simulink model "QuadcopterController"  (R2019a)
settings: Solver=VariableStepAuto  StartTime=0.0  StopTime=50  RelTol=1e-3
InitFcn:
  | parameters
values from neighbouring files (symbols this model uses):
  attitudeInit = [0;0;0]    [parameters.m]
  b = 5.9347e-06    [parameters.m]
  d = 1.2181e-07    [parameters.m]
  g = 9.81    [parameters.m]
  I = diag([Ix,Iy,Iz])    [parameters.m]
  Ix = 0.0073    [parameters.m]
  Iy = 0.0073    [parameters.m]
  Iz = 0.0117    [parameters.m]
  ks = 735    [parameters.m]
  Kth = b*lambda    [parameters.m]
  kxih = 0.7    [parameters.m]
  L = 0.17    [parameters.m]
  lambda = w0^2/u0    [parameters.m]
  m = 0.616    [parameters.m]
  omegaInit = [0;0;0]    [parameters.m]
  posInit = [0;0;0]    [parameters.m]
  tau = 1/200    (= 0.005)    [parameters.m]
  u0 = 0.49    [parameters.m]
  velInit = [0;0;0]    [parameters.m]
  w_n = 8    [parameters.m]
  wh_n = 2    [parameters.m]
  zeta = 0.7    [parameters.m]
settings Model: Creator=NGUYEN  LastModifiedBy=ASUS
settings SolverCC: ZeroCrossAlgorithm=Adaptive
settings OptimizationCC: LifeSpan=inf
settings DebuggingCC: IgnoredZcDiagnostic=none  ArithmeticOperatorsInVariantConditions=warning
settings CodeAppCC: StateflowObjectComments=on

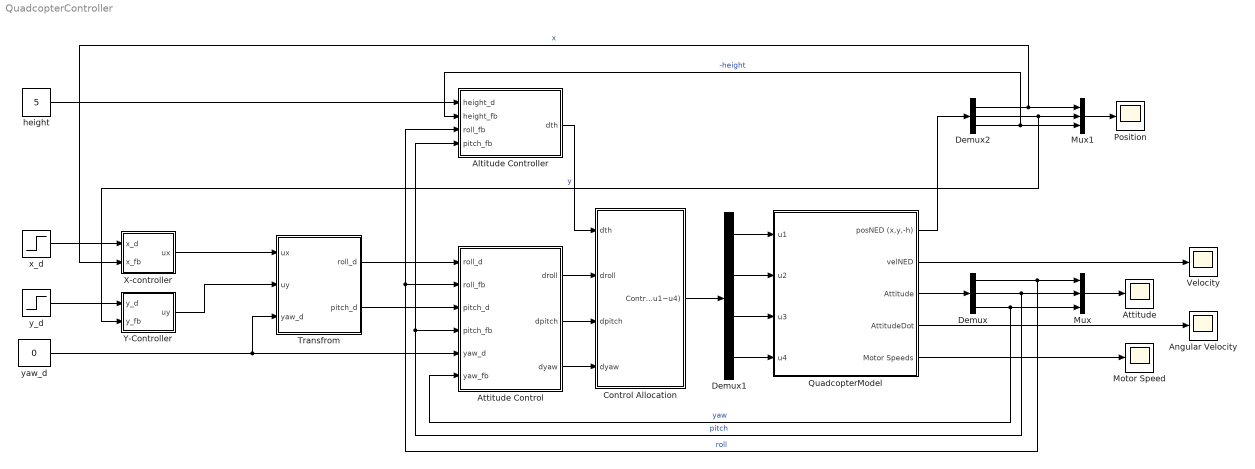
== system QuadcopterController ==
  Altitude Controller : Subsystem
  Angular Velocity : Scope
  Attitude : Scope
  Attitude Control : Subsystem
  Control Allocation : Subsystem
  Demux : Demux  Outputs=3
  Demux1 : Demux
  Demux2 : Demux  Outputs=3
  Motor Speed : Scope
  Mux : Mux  Inputs=3
  Mux1 : Mux  Inputs=3
  Position : Scope
  QuadcopterModel : Subsystem
  Transfrom : Subsystem
  Velocity : Scope
  X-controller : Subsystem
  Y-Controller : Subsystem
  height : Constant  Value=5
  x_d : Step  Time=0  After=5  SampleTime=0
  y_d : Step  Time=0  After=7  SampleTime=0
  yaw_d : Constant  Value=0
  wires:
  Demux/1 -> Mux/1, Altitude Controller/3(roll_fb), Attitude Control/2(roll_fb)  "roll"
  Demux/2 -> Mux/2, Altitude Controller/4(pitch_fb), Attitude Control/4(pitch_fb)  "pitch"
  Demux/3 -> Mux/3, Attitude Control/6(yaw_fb)  "yaw"
  Demux2/1 -> Mux1/1, X-controller/2(x_fb)  "x"
  Demux2/2 -> Mux1/2, Y-Controller/2(y_fb)  "y"
  Demux2/3 -> Mux1/3, Altitude Controller/2(height_fb)  "-height"
  Mux1/1 -> Position/1
  Mux/1 -> Attitude/1
  height/1 -> Altitude Controller/1(height_d)
  yaw_d/1 -> Attitude Control/5(yaw_d), Transfrom/3(yaw_d)
  X-controller/1(ux) -> Transfrom/1(ux)
  Y-Controller/1(uy) -> Transfrom/2(uy)
  y_d/1 -> Y-Controller/1(y_d)
  x_d/1 -> X-controller/1(x_d)
  Transfrom/1(roll_d) -> Attitude Control/1(roll_d)
  Transfrom/2(pitch_d) -> Attitude Control/3(pitch_d)
  Altitude Controller/1(dth) -> Control Allocation/1(dth)
  Attitude Control/1(droll) -> Control Allocation/2(droll)
  Attitude Control/2(dpitch) -> Control Allocation/3(dpitch)
  Attitude Control/3(dyaw) -> Control Allocation/4(dyaw)
  Control Allocation/1(Controller (u1~u4)) -> Demux1/1
  QuadcopterModel/1(posNED (x,y,-h)) -> Demux2/1
  QuadcopterModel/3(Attitude) -> Demux/1
  Demux1/1 -> QuadcopterModel/1(u1)
  Demux1/2 -> QuadcopterModel/2(u2)
  Demux1/3 -> QuadcopterModel/3(u3)
  Demux1/4 -> QuadcopterModel/4(u4)
  QuadcopterModel/4(AttitudeDot) -> Angular Velocity/1
  QuadcopterModel/2(velNED) -> Velocity/1
  QuadcopterModel/5(Motor Speeds) -> Motor Speed/1

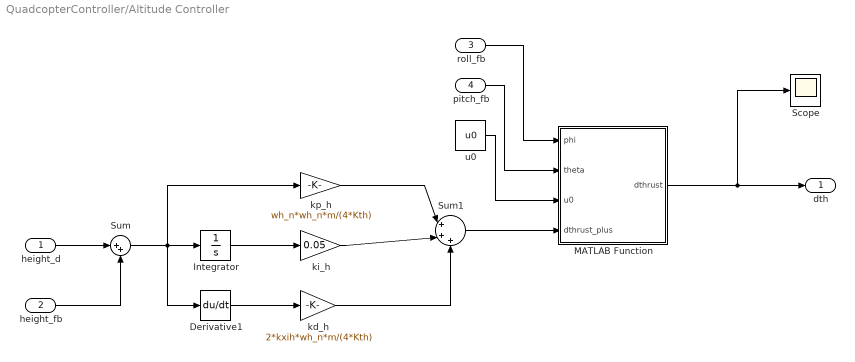
== system QuadcopterController/Altitude Controller ==
  height_d : Inport
  height_fb : Inport  Port=2
  roll_fb : Inport  Port=3
  pitch_fb : Inport  Port=4
  Derivative1 : Derivative
  Integrator : Integrator
  MATLAB Function : MATLAB Function  TreatAsAtomicUnit=on
  Scope : Scope
  Sum : Sum  Inputs=|++
  Sum1 : Sum  Inputs=|+++
  kd_h : Gain  Gain=2*kxih*wh_n*m/(4*Kth)
  ki_h : Gain  Gain=0.05
  kp_h : Gain  Gain=wh_n*wh_n*m/(4*Kth)
  u0 : Constant  Value=u0
  dth : Outport
  wires:
  Derivative1/1 -> kd_h/1
  height_d/1 -> Sum/1
  Sum/1 -> kp_h/1, Integrator/1, Derivative1/1
  height_fb/1 -> Sum/2
  Integrator/1 -> ki_h/1
  ki_h/1 -> Sum1/2
  kp_h/1 -> Sum1/1
  kd_h/1 -> Sum1/3
  Sum1/1 -> MATLAB Function/4(dthrust_plus)
  roll_fb/1 -> MATLAB Function/1(phi)
  pitch_fb/1 -> MATLAB Function/2(theta)
  MATLAB Function/1(dthrust) -> Scope/1, dth/1
  u0/1 -> MATLAB Function/3(u0)

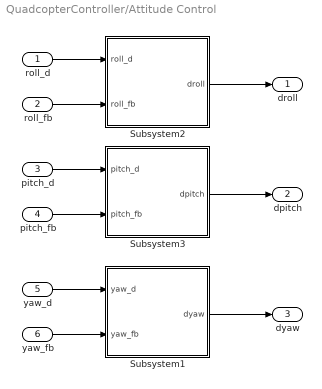
== system QuadcopterController/Attitude Control ==
  roll_d : Inport
  roll_fb : Inport  Port=2
  pitch_d : Inport  Port=3
  pitch_fb : Inport  Port=4
  yaw_d : Inport  Port=5
  yaw_fb : Inport  Port=6
  Subsystem1 : Subsystem
  Subsystem2 : Subsystem
  Subsystem3 : Subsystem
  droll : Outport
  dpitch : Outport  Port=2
  dyaw : Outport  Port=3
  wires:
  roll_d/1 -> Subsystem2/1(roll_d)
  Subsystem3/1(dpitch) -> dpitch/1
  roll_fb/1 -> Subsystem2/2(roll_fb)
  yaw_d/1 -> Subsystem1/1(yaw_d)
  Subsystem2/1(droll) -> droll/1
  pitch_d/1 -> Subsystem3/1(pitch_d)
  pitch_fb/1 -> Subsystem3/2(pitch_fb)
  yaw_fb/1 -> Subsystem1/2(yaw_fb)
  Subsystem1/1(dyaw) -> dyaw/1

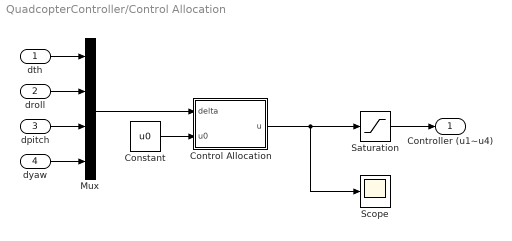
== system QuadcopterController/Control Allocation ==
  dth : Inport
  droll : Inport  Port=2
  dpitch : Inport  Port=3
  dyaw : Inport  Port=4
  Constant : Constant  Value=u0
  Control Allocation : MATLAB Function  TreatAsAtomicUnit=on
  Mux : Mux
  Saturation : Saturate  UpperLimit=1  LowerLimit=0  ZeroCross=off
  Scope : Scope
  Controller (u1~u4) : Outport
  wires:
  dth/1 -> Mux/1
  droll/1 -> Mux/2
  dpitch/1 -> Mux/3
  dyaw/1 -> Mux/4
  Constant/1 -> Control Allocation/2(u0)
  Mux/1 -> Control Allocation/1(delta)
  Control Allocation/1(u) -> Saturation/1, Scope/1
  Saturation/1 -> Controller (u1~u4)/1

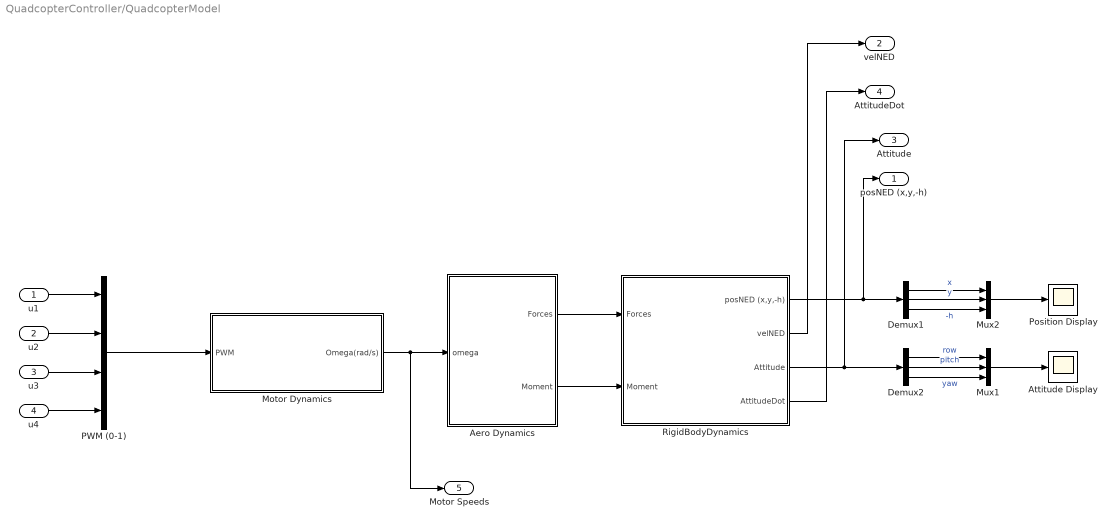
== system QuadcopterController/QuadcopterModel ==
  u1 : Inport
  u2 : Inport  Port=2
  u3 : Inport  Port=3
  u4 : Inport  Port=4
  Aero Dynamics : Subsystem
  Attitude Display : Scope
  Demux1 : Demux  Outputs=3
  Demux2 : Demux  Outputs=3
  Motor Dynamics : Subsystem
  Mux1 : Mux  Inputs=3
  Mux2 : Mux  Inputs=3
  PWM (0-1) : Mux
  Position Display : Scope
  RigidBodyDynamics : Subsystem
  posNED (x,y,-h) : Outport
  velNED : Outport  Port=2
  Attitude : Outport  Port=3
  AttitudeDot : Outport  Port=4
  Motor Speeds : Outport  Port=5
  wires:
  RigidBodyDynamics/2(velNED) -> velNED/1
  u2/1 -> PWM (0-1)/2
  Demux2/1 -> Mux1/1  "row"
  Demux2/2 -> Mux1/2  "pitch"
  Demux1/2 -> Mux2/2  "y"
  RigidBodyDynamics/1(posNED (x,y,-h)) -> Demux1/1, posNED (x,y,-h)/1
  Mux2/1 -> Position Display/1
  u4/1 -> PWM (0-1)/4
  Demux1/1 -> Mux2/1  "x"
  Motor Dynamics/1(Omega(rad/s)) -> Motor Speeds/1, Aero Dynamics/1(omega)
  Aero Dynamics/1(Forces) -> RigidBodyDynamics/1(Forces)
  Mux1/1 -> Attitude Display/1
  Demux2/3 -> Mux1/3  "yaw"
  Aero Dynamics/2(Moment) -> RigidBodyDynamics/2(Moment)
  Demux1/3 -> Mux2/3  "-h"
  RigidBodyDynamics/3(Attitude) -> Demux2/1, Attitude/1
  u3/1 -> PWM (0-1)/3
  RigidBodyDynamics/4(AttitudeDot) -> AttitudeDot/1
  u1/1 -> PWM (0-1)/1
  PWM (0-1)/1 -> Motor Dynamics/1(PWM)

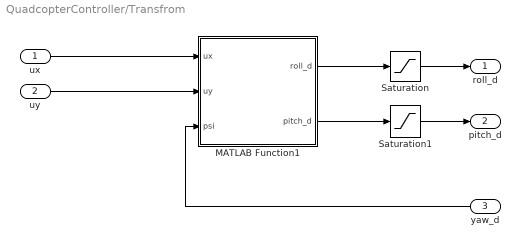
== system QuadcopterController/Transfrom ==
  ux : Inport
  uy : Inport  Port=2
  yaw_d : Inport  Port=3
  MATLAB Function1 : MATLAB Function  TreatAsAtomicUnit=on
  Saturation : Saturate  UpperLimit=pi/8  LowerLimit=-pi/8
  Saturation1 : Saturate  UpperLimit=pi/8  LowerLimit=-pi/8
  roll_d : Outport
  pitch_d : Outport  Port=2
  wires:
  MATLAB Function1/2(pitch_d) -> Saturation1/1
  MATLAB Function1/1(roll_d) -> Saturation/1
  ux/1 -> MATLAB Function1/1(ux)
  uy/1 -> MATLAB Function1/2(uy)
  yaw_d/1 -> MATLAB Function1/3(psi)
  Saturation/1 -> roll_d/1
  Saturation1/1 -> pitch_d/1

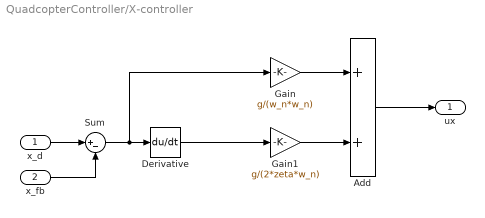
== system QuadcopterController/X-controller ==
  x_d : Inport
  x_fb : Inport  Port=2
  Add : Sum
  Derivative : Derivative
  "Gain  " : Gain  Gain=g/(w_n*w_n)
  Gain1 : Gain  Gain=g/(2*zeta*w_n)
  Sum : Sum  Inputs=|+-
  ux : Outport
  wires:
  Derivative/1 -> Gain1/1
  "Gain  "/1 -> Add/1
  Gain1/1 -> Add/2
  Sum/1 -> Derivative/1, "Gain  "/1
  x_d/1 -> Sum/1
  x_fb/1 -> Sum/2
  Add/1 -> ux/1

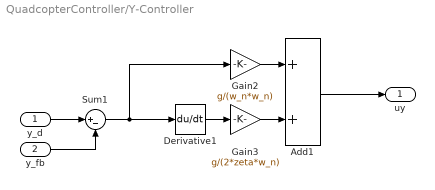
== system QuadcopterController/Y-Controller ==
  y_d : Inport
  y_fb : Inport  Port=2
  Add1 : Sum
  Derivative1 : Derivative
  Gain2 : Gain  Gain=g/(w_n*w_n)
  Gain3 : Gain  Gain=g/(2*zeta*w_n)
  Sum1 : Sum  Inputs=|+-
  uy : Outport
  wires:
  Gain3/1 -> Add1/2
  Sum1/1 -> Derivative1/1, Gain2/1
  Derivative1/1 -> Gain3/1
  Add1/1 -> uy/1
  Gain2/1 -> Add1/1
  y_d/1 -> Sum1/1
  y_fb/1 -> Sum1/2

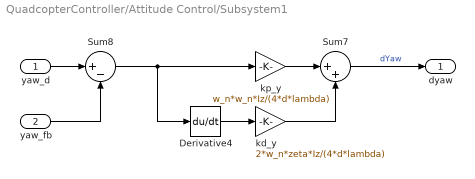
== system QuadcopterController/Attitude Control/Subsystem1 ==
  yaw_d : Inport
  yaw_fb : Inport  Port=2
  Derivative4 : Derivative
  Sum7 : Sum  Inputs=|++
  Sum8 : Sum  Inputs=|+-
  kd_y : Gain  Gain=2*w_n*zeta*Iz/(4*d*lambda)
  kp_y : Gain  Gain=w_n*w_n*Iz/(4*d*lambda)
  dyaw : Outport
  wires:
  kp_y/1 -> Sum7/1
  yaw_fb/1 -> Sum8/2
  kd_y/1 -> Sum7/2
  Derivative4/1 -> kd_y/1
  Sum7/1 -> dyaw/1  "dYaw"
  Sum8/1 -> kp_y/1, Derivative4/1
  yaw_d/1 -> Sum8/1

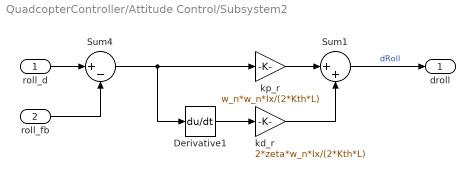
== system QuadcopterController/Attitude Control/Subsystem2 ==
  roll_d : Inport
  roll_fb : Inport  Port=2
  Derivative1 : Derivative
  Sum1 : Sum  Inputs=|++
  Sum4 : Sum  Inputs=|+-
  kd_r : Gain  Gain=2*zeta*w_n*Ix/(2*Kth*L)
  kp_r : Gain  Gain=w_n*w_n*Ix/(2*Kth*L)
  droll : Outport
  wires:
  Sum1/1 -> droll/1  "dRoll"
  Derivative1/1 -> kd_r/1
  Sum4/1 -> kp_r/1, Derivative1/1
  kd_r/1 -> Sum1/2
  kp_r/1 -> Sum1/1
  roll_fb/1 -> Sum4/2
  roll_d/1 -> Sum4/1

== system QuadcopterController/Attitude Control/Subsystem3 ==
  pitch_d : Inport
  pitch_fb : Inport  Port=2
  Derivative3 : Derivative
  Sum5 : Sum  Inputs=|++
  Sum6 : Sum  Inputs=|+-
  kd_p : Gain  Gain=2*zeta*w_n*Iy/(2*Kth*L)
  kp_p : Gain  Gain=w_n*w_n*Iy/(2*Kth*L)
  dpitch : Outport
  wires:
  kp_p/1 -> Sum5/1
  kd_p/1 -> Sum5/2
  Derivative3/1 -> kd_p/1
  pitch_d/1 -> Sum6/1
  Sum6/1 -> kp_p/1, Derivative3/1
  pitch_fb/1 -> Sum6/2
  Sum5/1 -> dpitch/1  "dPitch"

== system QuadcopterController/QuadcopterModel/Aero Dynamics ==
  omega : Inport
  Aero Dynamics : MATLAB Function  TreatAsAtomicUnit=on
  Constant : Constant  Value=d
  Constant1 : Constant  Value=b
  Constant2 : Constant  Value=L
  Forces : Outport
  Moment : Outport  Port=2
  wires:
  Aero Dynamics/2(Moments) -> Moment/1
  Constant/1 -> Aero Dynamics/4(d)
  Constant2/1 -> Aero Dynamics/2(L)
  Constant1/1 -> Aero Dynamics/3(b)
  Aero Dynamics/1(Forces) -> Forces/1
  omega/1 -> Aero Dynamics/1(omega)

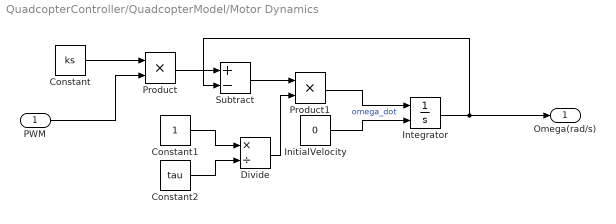
== system QuadcopterController/QuadcopterModel/Motor Dynamics ==
  PWM : Inport
  Constant : Constant  Value=ks
  Constant1 : Constant
  Constant2 : Constant  Value=tau
  Divide : Product  Inputs=*/
  InitialVelocity : Constant  Value=0
  Integrator : Integrator  InitialConditionSource=external
  Product : Product
  Product1 : Product
  Subtract : Sum  Inputs=+-
  Omega(rad/s) : Outport
  wires:
  Constant/1 -> Product/1
  Integrator/1 -> Omega(rad/s)/1, Subtract/2
  Divide/1 -> Product1/2
  Constant2/1 -> Divide/2
  Constant1/1 -> Divide/1
  Product1/1 -> Integrator/1  "omega_dot"
  InitialVelocity/1 -> Integrator/2
  Product/1 -> Subtract/1
  Subtract/1 -> Product1/1
  PWM/1 -> Product/2

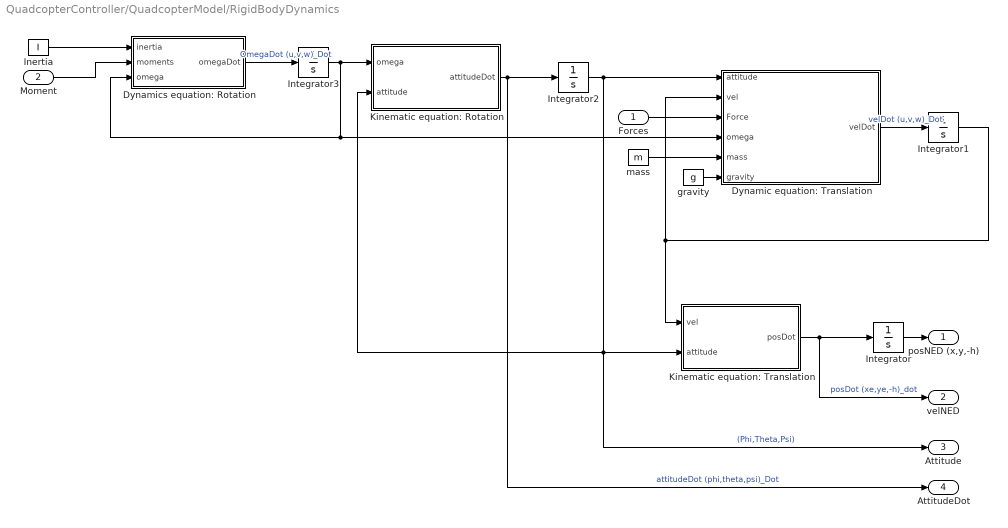
== system QuadcopterController/QuadcopterModel/RigidBodyDynamics ==
  Forces : Inport
  Moment : Inport  Port=2
  Dynamic equation: Translation : MATLAB Function  TreatAsAtomicUnit=on
  Dynamics equation: Rotation : MATLAB Function  TreatAsAtomicUnit=on
  Inertia : Constant  Value=I
  Integrator : Integrator  InitialCondition=posInit
  Integrator1 : Integrator  InitialCondition=velInit
  Integrator2 : Integrator  InitialCondition=attitudeInit
  Integrator3 : Integrator  InitialCondition=omegaInit
  Kinematic equation: Rotation : MATLAB Function  TreatAsAtomicUnit=on
  Kinematic equation: Translation : MATLAB Function  TreatAsAtomicUnit=on
  gravity : Constant  Value=g
  mass : Constant  Value=m
  posNED (x,y,-h) : Outport
  velNED : Outport  Port=2
  Attitude : Outport  Port=3
  AttitudeDot : Outport  Port=4
  wires:
  Integrator2/1 -> Kinematic equation: Translation/2(attitude), Attitude/1, Kinematic equation: Rotation/2(attitude), Dynamic equation: Translation/1(attitude)  "(Phi,Theta,Psi)"
  Dynamics equation: Rotation/1(omegaDot) -> Integrator3/1  "OmegaDot (u,v,w)_Dot"
  Integrator3/1 -> Kinematic equation: Rotation/1(omega), Dynamic equation: Translation/4(omega), Dynamics equation: Rotation/3(omega)
  Integrator/1 -> posNED (x,y,-h)/1
  Kinematic equation: Translation/1(posDot) -> Integrator/1, velNED/1  "posDot (xe,ye,-h)_dot"
  Kinematic equation: Rotation/1(attitudeDot) -> Integrator2/1, AttitudeDot/1  "attitudeDot (phi,theta,psi)_Dot"
  Inertia/1 -> Dynamics equation: Rotation/1(inertia)
  gravity/1 -> Dynamic equation: Translation/6(gravity)
  Moment/1 -> Dynamics equation: Rotation/2(moments)
  Forces/1 -> Dynamic equation: Translation/3(Force)
  mass/1 -> Dynamic equation: Translation/5(mass)
  Dynamic equation: Translation/1(velDot) -> Integrator1/1  "velDot (u,v,w)_Dot"
  Integrator1/1 -> Kinematic equation: Translation/1(vel), Dynamic equation: Translation/2(vel)

== matlab function QuadcopterController/QuadcopterModel/Aero Dynamics/Aero Dynamics ==
  data: Forces output; Moments output; omega input; L input; b input; d input
function [Forces,Moments] = fcn(omega, L, b, d)
% b: Cthurst, d: CDrag
Forces = [0;0;-b*(omega(1)^2 + omega(2)^2 + omega(3)^2 + omega(4)^2)];

Moments = [[L*b*(omega(4)^2 - omega(2)^2)];
    [L*b*(omega(1)^2 - omega(3)^2)];
    [d*(-omega(1)^2 + omega(2)^2 - omega(3)^2 + omega(4)^2)]];

% Drag = d*omega.^2;
% U1 = sum(b*omega.^2);
% U2 = L*b*(omega(4).^2-omega(2).^2);
% U3 = L*b*(omega(1).^2-omega(3).^2);
% U4 = -Drag(1)+Drag(2)-Drag(3)+Drag(4);
% Forces = [0;0;-U1];
% Moments = [U2;U3;U4];

== matlab function QuadcopterController/Control Allocation/Control Allocation ==
  data: delta input; u output; u0 input
function u = fcn(delta, u0)
% delta = dthrust,droll,dpitch,dyaw
% u = [u1 u2 u3 u4]
%     dthrust = delta(1);
%     droll = delta(2);
%     dpitch = delta(3);
%     dyaw = delta(4);
%     new_delta = [dthrust; droll; dpitch; dyaw];
    Control_Allocation_matrix = [[1 0 1 -1];[1 -1 0 1];[1 0 -1 -1];[1 1 0 1]];
    u = Control_Allocation_matrix * delta + [u0; u0; u0; u0];

== matlab function QuadcopterController/Altitude Controller/MATLAB Function ==
  data: phi input; dthrust output; theta input; u0 input; dthrust_plus input
function dthrust = fcn(phi, theta, u0,dthrust_plus)

dthrust = (u0+dthrust_plus)/(cos(phi)*cos(theta)) - u0;

== matlab function QuadcopterController/Transfrom/MATLAB Function1 ==
  data: ux input; roll_d output; uy input; psi input; pitch_d output
function [roll_d, pitch_d] = fcn(ux,uy,psi)
ux = -ux;
uy = -uy;
sin_roll_d = ux*sin(psi) - uy*cos(psi);
sin_roll_d = max(min(sin_roll_d,1),-1);
roll_d = asin(sin_roll_d);
sin_pitch_d = (ux*cos(psi)+uy*sin(psi))/cos(roll_d);
sin_pitch_d = max(min(sin_pitch_d,1),-1);
pitch_d = asin(sin_pitch_d);

== matlab function QuadcopterController/QuadcopterModel/RigidBodyDynamics/Dynamic equation: Translation ==
  data: attitude input; velDot output; vel input; Force input; omega input; mass input; gravity input
function velDot = fcn(attitude, vel, Force ,omega , mass, gravity)

phi = attitude(1);
theta = attitude(2);
psi = attitude(3);
% F1 = F(1);
% F2 = F(2);
% F3 = F(3);
% F4 = F(4);

%input: vel =[u;v;w], attitude = [phi;theta;psi], omega =[p;q;r], Force,
%gravity, mass, 

%output: velDot = [uDot, vDot, wDot]

velDot = [-gravity*sin(theta); gravity*sin(phi)*cos(theta); gravity*cos(phi)*cos(theta)] + Force/mass - cross(omega, vel);

== matlab function QuadcopterController/QuadcopterModel/RigidBodyDynamics/Dynamics equation: Rotation ==
  data: inertia input; omegaDot output; moments input; omega input
function omegaDot = fcn(inertia, moments, omega)
% input: omega: toc do goc cua, inertia: moments quan tinh, 
%moments: bien dieu khien moment cua dong co
% output: omegaDot
omegaDot = inertia^(-1)*(moments - cross(omega,inertia*omega));

== matlab function QuadcopterController/QuadcopterModel/RigidBodyDynamics/Kinematic equation: Rotation ==
  data: omega input; attitudeDot output; attitude input
function attitudeDot = fcn(omega, attitude)
phi = attitude(1);
theta = attitude(2);
psi = attitude(3);

W_BE = [[1, (sin(phi)*sin(theta))/cos(theta), (cos(phi)*sin(theta))/cos(theta)];
[0,                         cos(phi),                        -sin(phi)];
[0,              sin(phi)/cos(theta),              cos(phi)/cos(theta)]];

% input: omega =[p;q;r], attitude = [phi;theta;psi]
%output: attitudeDot = [phiDot;thetaDot;psiDot]
attitudeDot = W_BE*omega;

== matlab function QuadcopterController/QuadcopterModel/RigidBodyDynamics/Kinematic equation: Translation ==
  data: vel input; posDot output; attitude input
function posDot = fcn(vel, attitude)
phi = attitude(1);
theta = attitude(2);
psi = attitude(3);

R = [[cos(psi)*cos(theta), cos(psi)*sin(theta)*sin(phi) - cos(phi)*sin(psi), sin(psi)*sin(phi) + cos(psi)*cos(phi)*sin(theta)];
[cos(theta)*sin(psi), cos(psi)*cos(phi) + sin(psi)*sin(theta)*sin(phi), cos(phi)*sin(psi)*sin(theta) - cos(psi)*sin(phi)];
[       -sin(theta),                           cos(theta)*sin(phi),                           cos(theta)*cos(phi)]];

% Velocity output = [x_dot, y_dot, z_dot]
% input: vel =[u;v;w], attitude = [phi;theta;psi]
posDot = R*vel;
